simulink model "ADAPT_SDCAL_YesAccum_2Cyl_DA_11_30_2021"  (R2020b)
settings: Solver=ode15s  StartTime=0  StopTime=200  FixedStep=0.00125  MaxStep=0.00125  RelTol=1e-3  EnableMultiTasking=on
values from neighbouring files (symbols this model uses):
  Spring_const = -50    [Four_cyl_design_Param.m]    (also in Four_cyl_design_Param2.m = -200)
  Zero_Spr_F = 4    [Four_cyl_design_Param.m]    (also in Four_cyl_design_Param2.m)
undefined symbols (not defined in the file or in its folder): body, DiscIntNeverNeededParam, geometry, hydroData, pto
libraries: fl_lib x274, nesl_utility x158, sh_lib x128, WECSim_Lib x4
(part 3 of 11)

== system ADAPT_SDCAL_YesAccum_2Cyl_DA_11_30_2021/PTO-Sim - Crankshaft DA 4 Cylinders Case 5 good extra Short cylinders Comp Off/Cylinder 1 ==
  Crank Radius : Inport
  Spool Radius : Inport  Port=2
  Angle Displacement : Inport  Port=3
  Crank Init Angle : Inport  Port=4
  Ext Control Input : Inport  Port=5
  Comp Control Input : Inport  Port=6
  Crank Torque [Nm] : Product
  Crank Torque [Nm] Sensor : Scope
  Cyl1 Force Sensor : Scope
  Cylinder 1 to PTO Force convert : Subsystem
  Hydraulic cylinder and valves : Subsystem
  Ideal Translational Motion Sensor : fl_lib/Mechanical/Mechanical Sensors/Ideal Translational Motion Sensor  offset=0 m
  Mass : fl_lib/Mechanical/Translational Elements/Mass  mass=1 kg  v_specify=off  v_priority=High  v=0 m/s  v_nominal_specify=off  v_nominal_unit=m/s  v_nominal_value=1  f_specify=off  f_priority=None  f=0 N  f_nominal_specify=off  f_nominal_unit=N  f_nominal_value=1
  PTO Force Cyl 1 Sensor : Scope
  Slider-Crank : fl_lib/Mechanical/Mechanisms/Slider-Crank  crank=3.136 in  rod=7 in  inertia=0.01 kg*m^2  k=1e6 N/m  b=0.0001 N/(m/s)  theta_specify=on  theta_priority=High  theta=pi / 2 rad  theta_nominal_specify=off  theta_nominal_unit=rad  theta_nominal_value=1  w_specify=off  w_priority=Low  w=0 rad/s  w_nominal_specify=off  w_nominal_unit=rad/s  w_nominal_value=1
      settings: SourceProductBaseCode=SS  InternalSimscapePortConfiguration="{\"Bottom\":[],\"Left\":[{\"id\":\"C\",\"label\":\"C\",\"type\":\"foundation.mechanical.rotational.rotational\"}],\"Right\":[{\"id\":\"S\",\"label\":\"S\",\"type\":\"foundation.mechanical.translational.translational\"}],\"Top\":[]}"
  Theta sensor : Scope
  sin(theta) sensor : Scope
  Angular Vel Source : PMIOPort  Side=Left
  Flow Out : PMIOPort  Port=2  Side=Left
  Flow In : PMIOPort  Port=3  Side=Left
  PTO Force : Outport
  wires:
  Crank Torque [Nm]/1 -> Crank Torque [Nm] Sensor/1
  Hydraulic cylinder and valves/1(Force Out) -> Cylinder 1 to PTO Force convert/5(Cylinder Force), Cyl1 Force Sensor/1
  Crank Radius/1 -> Cylinder 1 to PTO Force convert/1(Crank radius), Crank Torque [Nm]/1
  Cylinder 1 to PTO Force convert/3(PTO Force Cyl) -> PTO Force/1, Crank Torque [Nm]/2, PTO Force Cyl 1 Sensor/1
  Cylinder 1 to PTO Force convert/2(sing(theta)) -> sin(theta) sensor/1
  Spool Radius/1 -> Cylinder 1 to PTO Force convert/4(Spool radius)
  Cylinder 1 to PTO Force convert/1(Theta) -> Theta sensor/1
  Crank Init Angle/1 -> Cylinder 1 to PTO Force convert/2(Crank initial angle)
  Angle Displacement/1 -> Cylinder 1 to PTO Force convert/3(Angle disp)
  Ext Control Input/1 -> Hydraulic cylinder and valves/1(Ext Control Input)
  Comp Control Input/1 -> Hydraulic cylinder and valves/2(Comp Control Input)
  connections:
  Hydraulic cylinder and valves/LConn1 -- Ideal Translational Motion Sensor/RConn2
  Mass/LConn1 -- Ideal Translational Motion Sensor/RConn1
  Slider-Crank/RConn1 -- Ideal Translational Motion Sensor/LConn1
  Slider-Crank/LConn1 -- Angular Vel Source/RConn1
  Hydraulic cylinder and valves/LConn3 -- Flow In/RConn1
  Hydraulic cylinder and valves/LConn2 -- Flow Out/RConn1

== system ADAPT_SDCAL_YesAccum_2Cyl_DA_11_30_2021/PTO-Sim - Crankshaft DA 4 Cylinders Case 5 good extra Short cylinders Comp Off/Cylinder 2 ==
  Crank Radius : Inport
  Spool Radius : Inport  Port=2
  Angle Displacement : Inport  Port=3
  Crank Init Angle : Inport  Port=4
  Ext Control Input : Inport  Port=5
  Comp Control Input : Inport  Port=6
  Crank Torque [Nm] : Product
  Crank Torque [Nm] Sensor : Scope
  Cyl1 Force Sensor : Scope
  Cylinder 1 to PTO Force convert : Subsystem
  Hydraulic cylinder and valves : Subsystem
  Ideal Translational Motion Sensor : fl_lib/Mechanical/Mechanical Sensors/Ideal Translational Motion Sensor  offset=0 m
  Mass : fl_lib/Mechanical/Translational Elements/Mass  mass=1 kg  v_specify=off  v_priority=High  v=0 m/s  v_nominal_specify=off  v_nominal_unit=m/s  v_nominal_value=1  f_specify=off  f_priority=None  f=0 N  f_nominal_specify=off  f_nominal_unit=N  f_nominal_value=1
  PTO Force Cyl 1 Sensor : Scope
  Slider-Crank : fl_lib/Mechanical/Mechanisms/Slider-Crank  crank=3.136 in  rod=7 in  inertia=0.01 kg*m^2  k=1e6 N/m  b=0.0001 N/(m/s)  theta_specify=on  theta_priority=High  theta=0 rad  theta_nominal_specify=off  theta_nominal_unit=rad  theta_nominal_value=1  w_specify=off  w_priority=Low  w=0 rad/s  w_nominal_specify=off  w_nominal_unit=rad/s  w_nominal_value=1
      settings: SourceProductBaseCode=SS  InternalSimscapePortConfiguration="{\"Bottom\":[],\"Left\":[{\"id\":\"C\",\"label\":\"C\",\"type\":\"foundation.mechanical.rotational.rotational\"}],\"Right\":[{\"id\":\"S\",\"label\":\"S\",\"type\":\"foundation.mechanical.translational.translational\"}],\"Top\":[]}"
  Theta sensor : Scope
  sin(theta) sensor : Scope
  Angular Vel Source : PMIOPort  Side=Left
  Flow Out : PMIOPort  Port=2  Side=Left
  Flow In : PMIOPort  Port=3  Side=Left
  PTO Force : Outport
  wires:
  Crank Torque [Nm]/1 -> Crank Torque [Nm] Sensor/1
  Hydraulic cylinder and valves/1(Force Out) -> Cylinder 1 to PTO Force convert/5(Cylinder Force), Cyl1 Force Sensor/1
  Crank Radius/1 -> Cylinder 1 to PTO Force convert/1(Crank radius), Crank Torque [Nm]/1
  Cylinder 1 to PTO Force convert/3(PTO Force Cyl) -> PTO Force/1, Crank Torque [Nm]/2, PTO Force Cyl 1 Sensor/1
  Cylinder 1 to PTO Force convert/2(sing(theta)) -> sin(theta) sensor/1
  Spool Radius/1 -> Cylinder 1 to PTO Force convert/4(Spool radius)
  Cylinder 1 to PTO Force convert/1(Theta) -> Theta sensor/1
  Crank Init Angle/1 -> Cylinder 1 to PTO Force convert/2(Crank initial angle)
  Angle Displacement/1 -> Cylinder 1 to PTO Force convert/3(Angle disp)
  Ext Control Input/1 -> Hydraulic cylinder and valves/1(Ext Control Input)
  Comp Control Input/1 -> Hydraulic cylinder and valves/2(Comp Control Input)
  connections:
  Hydraulic cylinder and valves/LConn1 -- Ideal Translational Motion Sensor/RConn2
  Mass/LConn1 -- Ideal Translational Motion Sensor/RConn1
  Slider-Crank/RConn1 -- Ideal Translational Motion Sensor/LConn1
  Slider-Crank/LConn1 -- Angular Vel Source/RConn1
  Hydraulic cylinder and valves/LConn3 -- Flow In/RConn1
  Hydraulic cylinder and valves/LConn2 -- Flow Out/RConn1

== system ADAPT_SDCAL_YesAccum_2Cyl_DA_11_30_2021/PTO-Sim - Crankshaft DA 4 Cylinders Case 5 good extra Short cylinders Comp Off/Cylinder 3 ==
  Crank Radius : Inport
  Spool Radius : Inport  Port=2
  Angle Displacement : Inport  Port=3
  Crank Init Angle : Inport  Port=4
  Ext Control Input : Inport  Port=5
  Comp Control Input : Inport  Port=6
  Crank Torque [Nm] : Product
  Crank Torque [Nm] Sensor : Scope
  Cyl1 Force Sensor : Scope
  Cylinder 1 to PTO Force convert : Subsystem
  Hydraulic cylinder and valves : Subsystem
  Ideal Translational Motion Sensor : fl_lib/Mechanical/Mechanical Sensors/Ideal Translational Motion Sensor  offset=0 m
  Mass : fl_lib/Mechanical/Translational Elements/Mass  mass=1 kg  v_specify=off  v_priority=High  v=0 m/s  v_nominal_specify=off  v_nominal_unit=m/s  v_nominal_value=1  f_specify=off  f_priority=None  f=0 N  f_nominal_specify=off  f_nominal_unit=N  f_nominal_value=1
  PTO Force Cyl 1 Sensor : Scope
  Slider-Crank : fl_lib/Mechanical/Mechanisms/Slider-Crank  crank=3.136 in  rod=7 in  inertia=0.01 kg*m^2  k=1e6 N/m  b=0.0001 N/(m/s)  theta_specify=on  theta_priority=High  theta=3*pi/2 rad  theta_nominal_specify=off  theta_nominal_unit=rad  theta_nominal_value=1  w_specify=off  w_priority=Low  w=0 rad/s  w_nominal_specify=off  w_nominal_unit=rad/s  w_nominal_value=1
      settings: SourceProductBaseCode=SS  InternalSimscapePortConfiguration="{\"Bottom\":[],\"Left\":[{\"id\":\"C\",\"label\":\"C\",\"type\":\"foundation.mechanical.rotational.rotational\"}],\"Right\":[{\"id\":\"S\",\"label\":\"S\",\"type\":\"foundation.mechanical.translational.translational\"}],\"Top\":[]}"
  Theta sensor : Scope
  sin(theta) sensor : Scope
  Angular Vel Source : PMIOPort  Side=Left
  Flow Out : PMIOPort  Port=2  Side=Left
  Flow In : PMIOPort  Port=3  Side=Left
  PTO Force : Outport
  wires:
  Crank Torque [Nm]/1 -> Crank Torque [Nm] Sensor/1
  Hydraulic cylinder and valves/1(Force Out) -> Cylinder 1 to PTO Force convert/5(Cylinder Force), Cyl1 Force Sensor/1
  Crank Radius/1 -> Cylinder 1 to PTO Force convert/1(Crank radius), Crank Torque [Nm]/1
  Cylinder 1 to PTO Force convert/3(PTO Force Cyl) -> PTO Force/1, Crank Torque [Nm]/2, PTO Force Cyl 1 Sensor/1
  Cylinder 1 to PTO Force convert/2(sing(theta)) -> sin(theta) sensor/1
  Spool Radius/1 -> Cylinder 1 to PTO Force convert/4(Spool radius)
  Cylinder 1 to PTO Force convert/1(Theta) -> Theta sensor/1
  Crank Init Angle/1 -> Cylinder 1 to PTO Force convert/2(Crank initial angle)
  Angle Displacement/1 -> Cylinder 1 to PTO Force convert/3(Angle disp)
  Ext Control Input/1 -> Hydraulic cylinder and valves/1(Ext Control Input)
  Comp Control Input/1 -> Hydraulic cylinder and valves/2(Comp Control Input)
  connections:
  Hydraulic cylinder and valves/LConn1 -- Ideal Translational Motion Sensor/RConn2
  Mass/LConn1 -- Ideal Translational Motion Sensor/RConn1
  Slider-Crank/RConn1 -- Ideal Translational Motion Sensor/LConn1
  Slider-Crank/LConn1 -- Angular Vel Source/RConn1
  Hydraulic cylinder and valves/LConn3 -- Flow In/RConn1
  Hydraulic cylinder and valves/LConn2 -- Flow Out/RConn1

== system ADAPT_SDCAL_YesAccum_2Cyl_DA_11_30_2021/PTO-Sim - Crankshaft DA 4 Cylinders Case 5 good extra Short cylinders Comp Off/Cylinder 4 ==
  Crank Radius : Inport
  Spool Radius : Inport  Port=2
  Angle Displacement : Inport  Port=3
  Crank Init Angle : Inport  Port=4
  Ext Control Input : Inport  Port=5
  Comp Control Input : Inport  Port=6
  Crank Torque [Nm] : Product
  Crank Torque [Nm] Sensor : Scope
  Cyl1 Force Sensor : Scope
  Cylinder 1 to PTO Force convert : Subsystem
  Hydraulic cylinder and valves : Subsystem
  Ideal Translational Motion Sensor : fl_lib/Mechanical/Mechanical Sensors/Ideal Translational Motion Sensor  offset=0 m
  Mass : fl_lib/Mechanical/Translational Elements/Mass  mass=1 kg  v_specify=off  v_priority=High  v=0 m/s  v_nominal_specify=off  v_nominal_unit=m/s  v_nominal_value=1  f_specify=off  f_priority=None  f=0 N  f_nominal_specify=off  f_nominal_unit=N  f_nominal_value=1
  PTO Force Cyl 1 Sensor : Scope
  Slider-Crank : fl_lib/Mechanical/Mechanisms/Slider-Crank  crank=3.136 in  rod=7 in  inertia=0.01 kg*m^2  k=1e6 N/m  b=0.0001 N/(m/s)  theta_specify=on  theta_priority=High  theta=pi rad  theta_nominal_specify=off  theta_nominal_unit=rad  theta_nominal_value=1  w_specify=off  w_priority=Low  w=0 rad/s  w_nominal_specify=off  w_nominal_unit=rad/s  w_nominal_value=1
      settings: SourceProductBaseCode=SS  InternalSimscapePortConfiguration="{\"Bottom\":[],\"Left\":[{\"id\":\"C\",\"label\":\"C\",\"type\":\"foundation.mechanical.rotational.rotational\"}],\"Right\":[{\"id\":\"S\",\"label\":\"S\",\"type\":\"foundation.mechanical.translational.translational\"}],\"Top\":[]}"
  Theta sensor : Scope
  sin(theta) sensor : Scope
  Angular Vel Source : PMIOPort  Side=Left
  Flow Out : PMIOPort  Port=2  Side=Left
  Flow In : PMIOPort  Port=3  Side=Left
  PTO Force : Outport
  wires:
  Crank Torque [Nm]/1 -> Crank Torque [Nm] Sensor/1
  Hydraulic cylinder and valves/1(Force Out) -> Cylinder 1 to PTO Force convert/5(Cylinder Force), Cyl1 Force Sensor/1
  Crank Radius/1 -> Cylinder 1 to PTO Force convert/1(Crank radius), Crank Torque [Nm]/1
  Cylinder 1 to PTO Force convert/3(PTO Force Cyl) -> PTO Force/1, Crank Torque [Nm]/2, PTO Force Cyl 1 Sensor/1
  Cylinder 1 to PTO Force convert/2(sing(theta)) -> sin(theta) sensor/1
  Spool Radius/1 -> Cylinder 1 to PTO Force convert/4(Spool radius)
  Cylinder 1 to PTO Force convert/1(Theta) -> Theta sensor/1
  Crank Init Angle/1 -> Cylinder 1 to PTO Force convert/2(Crank initial angle)
  Angle Displacement/1 -> Cylinder 1 to PTO Force convert/3(Angle disp)
  Ext Control Input/1 -> Hydraulic cylinder and valves/1(Ext Control Input)
  Comp Control Input/1 -> Hydraulic cylinder and valves/2(Comp Control Input)
  connections:
  Hydraulic cylinder and valves/LConn1 -- Ideal Translational Motion Sensor/RConn2
  Mass/LConn1 -- Ideal Translational Motion Sensor/RConn1
  Slider-Crank/RConn1 -- Ideal Translational Motion Sensor/LConn1
  Slider-Crank/LConn1 -- Angular Vel Source/RConn1
  Hydraulic cylinder and valves/LConn3 -- Flow In/RConn1
  Hydraulic cylinder and valves/LConn2 -- Flow Out/RConn1

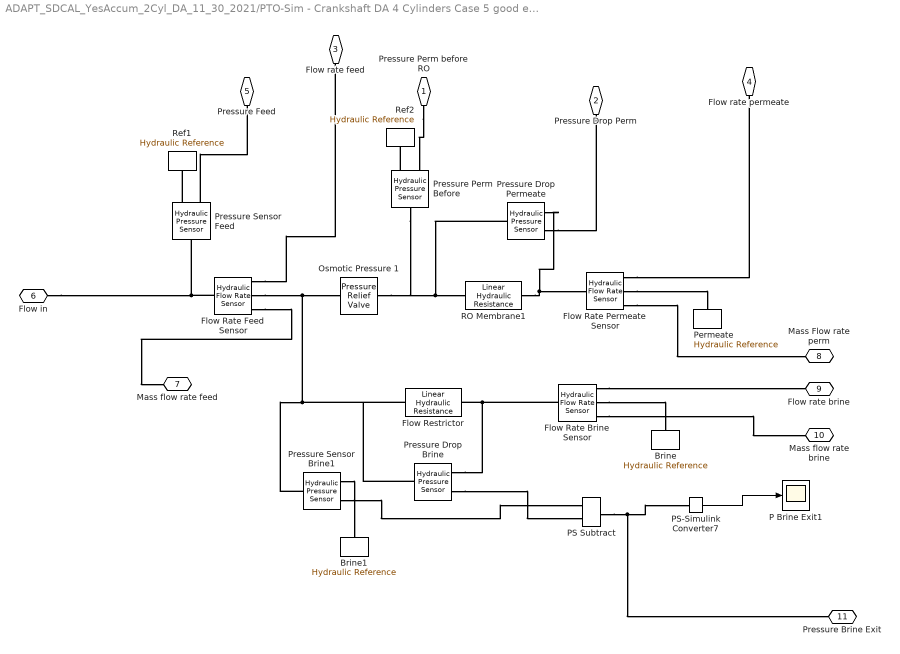
== system ADAPT_SDCAL_YesAccum_2Cyl_DA_11_30_2021/PTO-Sim - Crankshaft DA 4 Cylinders Case 5 good extra Short cylinders Comp Off/RO Membrane ==
  " Flow Rate Feed Sensor" : fl_lib/Hydraulic/Hydraulic Sensors/Hydraulic Flow Rate Sensor
  Brine : fl_lib/Hydraulic/Hydraulic Elements/Hydraulic Reference
  Brine1 : fl_lib/Hydraulic/Hydraulic Elements/Hydraulic Reference
  Flow Rate Brine Sensor : fl_lib/Hydraulic/Hydraulic Sensors/Hydraulic Flow Rate Sensor
  Flow Rate Permeate Sensor : fl_lib/Hydraulic/Hydraulic Sensors/Hydraulic Flow Rate Sensor
  Flow Restrictor : fl_lib/Hydraulic/Hydraulic Elements/Linear Hydraulic Resistance  resistance=(0.90) * ( 1/((3.812*10^-12)*(7.4 ) ) ) Pa/(m^3/s)  q_specify=off  q_priority=None  q=0.001 m^3/s  q_nominal_specify=off  q_nominal_unit=m^3/s  q_nominal_value=1  p_specify=off  p_priority=None  p=0 Pa  p_nominal_specify=off  p_nominal_unit=Pa  p_nominal_value=1
      settings: SourceProductBaseCode=SS  InternalSimscapePortConfiguration="{\"Bottom\":[],\"Left\":[{\"id\":\"A\",\"label\":\"A\",\"type\":\"foundation.hydraulic.hydraulic\"}],\"Right\":[{\"id\":\"B\",\"label\":\"B\",\"type\":\"foundation.hydraulic.hydraulic\"}],\"Top\":[]}"
  Osmotic Pressure 1 : sh_lib/Valves/Pressure Control Valves/Pressure Relief Valve  valve_area_spec=1  p_diff_TLU=[30.15e5 : 15e3 : 31.35e5] Pa  area_TLU=[1 : 1 : 9] .* 1e-5 m^2  area_max=10*pi*(0.75/2)^2 in^2  pres_set=30 bar  reg_range=2 bar  C_d=0.7  A_leak=1e-12 m^2  lam_spec=1  B_lam=0.999  Re_cr=12  dynamic=0  tau=0.1 s  area_init=1e-12 m^2
      settings: SourceProductBaseCode=SH  InternalSimscapePortConfiguration="{\"Bottom\":[],\"Left\":[{\"id\":\"A\",\"label\":\"A\",\"type\":\"foundation.hydraulic.hydraulic\"}],\"Right\":[{\"id\":\"B\",\"label\":\"B\",\"type\":\"foundation.hydraulic.hydraulic\"}],\"Top\":[]}"
  P Brine Exit1 : Scope
  PS Subtract : fl_lib/Physical Signals/Functions/PS Subtract
  PS-Simulink Converter7 : nesl_utility/PS-Simulink Converter  PhysicalDomain=network_engine_domain  SubClassName=ps_output  LeftPortType=input  RightPortType=output  PseudoPeriodic=off  Frequencies=[]  Unit=inherit  AffineConversion=off
  Permeate : fl_lib/Hydraulic/Hydraulic Elements/Hydraulic Reference
  Pressure Drop Brine : fl_lib/Hydraulic/Hydraulic Sensors/Hydraulic Pressure Sensor
  Pressure Drop Permeate : fl_lib/Hydraulic/Hydraulic Sensors/Hydraulic Pressure Sensor
  Pressure Perm Before : fl_lib/Hydraulic/Hydraulic Sensors/Hydraulic Pressure Sensor
  Pressure Sensor Brine1 : fl_lib/Hydraulic/Hydraulic Sensors/Hydraulic Pressure Sensor
  Pressure Sensor Feed : fl_lib/Hydraulic/Hydraulic Sensors/Hydraulic Pressure Sensor
  RO Membrane1 : fl_lib/Hydraulic/Hydraulic Elements/Linear Hydraulic Resistance  resistance=1/((3.812*10^-12)*(7.4 ) ) Pa/(m^3/s)  q_specify=off  q_priority=None  q=0.001 m^3/s  q_nominal_specify=off  q_nominal_unit=m^3/s  q_nominal_value=1  p_specify=off  p_priority=None  p=0 Pa  p_nominal_specify=off  p_nominal_unit=Pa  p_nominal_value=1
      settings: SourceProductBaseCode=SS  InternalSimscapePortConfiguration="{\"Bottom\":[],\"Left\":[{\"id\":\"A\",\"label\":\"A\",\"type\":\"foundation.hydraulic.hydraulic\"}],\"Right\":[{\"id\":\"B\",\"label\":\"B\",\"type\":\"foundation.hydraulic.hydraulic\"}],\"Top\":[]}"
  Ref1 : fl_lib/Hydraulic/Hydraulic Elements/Hydraulic Reference
  Ref2 : fl_lib/Hydraulic/Hydraulic Elements/Hydraulic Reference
  Pressure Perm before RO : PMIOPort  Side=Right
  Pressure Drop Perm : PMIOPort  Port=2  Side=Right
  Flow rate feed : PMIOPort  Port=3  Side=Right
  Flow rate permeate : PMIOPort  Port=4  Side=Right
  Pressure Feed : PMIOPort  Port=5  Side=Right
  Flow in : PMIOPort  Port=6  Side=Left
  Mass flow rate feed : PMIOPort  Port=7  Side=Right
  Mass Flow rate perm : PMIOPort  Port=8  Side=Right
  Flow rate brine : PMIOPort  Port=9  Side=Right
  Mass flow rate brine : PMIOPort  Port=10  Side=Right
  Pressure Brine Exit : PMIOPort  Port=11  Side=Right
  wires:
  PS-Simulink Converter7/1 -> P Brine Exit1/1
  connections:
  RO Membrane1/RConn1 -- Pressure Drop Permeate/RConn1 -- Flow Rate Permeate Sensor/LConn1
  " Flow Rate Feed Sensor"/RConn2 -- Pressure Sensor Brine1/LConn1 -- Pressure Drop Brine/LConn1 -- Flow Restrictor/LConn1 -- Osmotic Pressure 1/LConn1
  Pressure Drop Permeate/LConn1 -- RO Membrane1/LConn1 -- Osmotic Pressure 1/RConn1 -- Pressure Perm Before/LConn1
  Pressure Perm Before/RConn1 -- Ref2/LConn1
  Flow Rate Brine Sensor/LConn1 -- Pressure Drop Brine/RConn1 -- Flow Restrictor/RConn1
  " Flow Rate Feed Sensor"/LConn1 -- Pressure Sensor Feed/LConn1 -- Flow in/RConn1
  Flow Rate Permeate Sensor/RConn2 -- Permeate/LConn1
  Pressure Sensor Brine1/RConn1 -- Brine1/LConn1
  " Flow Rate Feed Sensor"/RConn1 -- Flow rate feed/RConn1
  PS Subtract/RConn1 -- Pressure Brine Exit/RConn1 -- PS-Simulink Converter7/LConn1
  Pressure Sensor Feed/RConn2 -- Pressure Feed/RConn1
  Flow Rate Brine Sensor/RConn2 -- Brine/LConn1
  Pressure Sensor Feed/RConn1 -- Ref1/LConn1
  Flow Rate Permeate Sensor/RConn1 -- Flow rate permeate/RConn1
  Pressure Perm before RO/RConn1 -- Pressure Perm Before/RConn2
  Pressure Drop Brine/RConn2 -- PS Subtract/LConn2
  Pressure Sensor Brine1/RConn2 -- PS Subtract/LConn1
  Pressure Drop Permeate/RConn2 -- Pressure Drop Perm/RConn1
  " Flow Rate Feed Sensor"/RConn3 -- Mass flow rate feed/RConn1
  Flow Rate Permeate Sensor/RConn3 -- Mass Flow rate perm/RConn1
  Flow Rate Brine Sensor/RConn1 -- Flow rate brine/RConn1
  Flow Rate Brine Sensor/RConn3 -- Mass flow rate brine/RConn1

== system ADAPT_SDCAL_YesAccum_2Cyl_DA_11_30_2021/PTO-Sim - Crankshaft DA 4 Cylinders Case 5 good extra Short cylinders Comp Off/Water Quality Block ==
  A_w/Bs : fl_lib/Physical Signals/Functions/PS Gain  gain=3.812*10^(-12)/(6.986*10^(-8))
  C_m : fl_lib/Physical Signals/Sources/PS Constant  constant=35000
  Constant : Constant  Value=0
  Cp : Scope  NumInputPorts=2
  Divide : Product
  If : If
  If Action Perm Flow  > 0 : Subsystem  TreatAsAtomicUnit=on
  If Action Subsystem1 : Subsystem  TreatAsAtomicUnit=on
  P Permeate Exit : Scope
  PS Add : fl_lib/Physical Signals/Functions/PS Add
  PS Constant : fl_lib/Physical Signals/Sources/PS Constant  constant=1 Pa
  PS Divide : fl_lib/Physical Signals/Functions/PS Divide
      settings: SourceProductBaseCode=SS
  PS Subtract1 : fl_lib/Physical Signals/Functions/PS Subtract
  PS-Simulink Converter{5..6,8..11} (6 alike) : nesl_utility/PS-Simulink Converter  PhysicalDomain=network_engine_domain  SubClassName=ps_output  LeftPortType=input  RightPortType=output  PseudoPeriodic=off  Frequencies=[]  Unit=inherit  AffineConversion=off
  Permeate Cp*Flow : Scope
  Recov Ratio : fl_lib/Physical Signals/Functions/PS Divide
      settings: SourceProductBaseCode=SS
  Recov Ratio % : Scope
  Pressure Perm Before : PMIOPort  Side=Left
  Pressure Dop Permeate : PMIOPort  Port=2  Side=Left
  Flow rate feed sensor : PMIOPort  Port=3  Side=Left
  Flow rate permeate : PMIOPort  Port=4  Side=Left
  wires:
  If Action Perm Flow  > 0/1(Out1) -> Cp/2
  Divide/1 -> Permeate Cp*Flow/1
  If/1 -> If Action Perm Flow  > 0/Action
  If Action Subsystem1/1(Out1) -> Cp/1
  If/2 -> If Action Subsystem1/Action
  PS-Simulink Converter10/1 -> Divide/1
  PS-Simulink Converter9/1 -> If/1
  PS-Simulink Converter8/1 -> P Permeate Exit/1
  PS-Simulink Converter6/1 -> Recov Ratio %/1
  PS-Simulink Converter11/1 -> Divide/2
  Constant/1 -> If Action Subsystem1/1(In1)
  PS-Simulink Converter5/1 -> If Action Perm Flow  > 0/1(In1)
  connections:
  A_w/Bs/LConn1 -- PS-Simulink Converter9/LConn1 -- PS Subtract1/LConn1 -- Pressure Perm Before/RConn1
  PS Divide/RConn1 -- PS-Simulink Converter5/LConn1 -- PS-Simulink Converter10/LConn1
  Recov Ratio/RConn1 -- PS-Simulink Converter6/LConn1
  PS Constant/RConn1 -- PS Add/LConn2
  Recov Ratio/LConn1 -- PS-Simulink Converter11/LConn1 -- Flow rate permeate/RConn1
  PS Subtract1/RConn1 -- PS-Simulink Converter8/LConn1
  PS Add/LConn1 -- A_w/Bs/RConn1
  C_m/RConn1 -- PS Divide/LConn1
  PS Divide/LConn2 -- PS Add/RConn1
  Flow rate feed sensor/RConn1 -- Recov Ratio/LConn2
  Pressure Dop Permeate/RConn1 -- PS Subtract1/LConn2

== system ADAPT_SDCAL_YesAccum_2Cyl_DA_11_30_2021/PTO-Sim - Crankshaft DA 4 Cylinders - 1 RO membrane/2 cylinders and valves/Cylinder 1 ==
  Crank Radius : Inport
  Spool Radius : Inport  Port=2
  Angle Displacement : Inport  Port=3
  Crank Init Angle : Inport  Port=4
  Ext Control Input : Inport  Port=5
  Comp Control Input : Inport  Port=6
  Crank Torque [Nm] : Product
  Crank Torque [Nm] Sensor : Scope
  Cyl1 Force Sensor : Scope
  Cylinder 1 to PTO Force convert : Subsystem
  Hydraulic cylinder and valves : Subsystem
  Ideal Translational Motion Sensor : fl_lib/Mechanical/Mechanical Sensors/Ideal Translational Motion Sensor  offset=0 m
  Mass : fl_lib/Mechanical/Translational Elements/Mass  mass=1 kg  num_ports=foundation.enum.numPorts2.one  v_specify=off  v_priority=High  v=0 m/s  v_nominal_specify=off  v_nominal_unit=m/s  v_nominal_value=1  f_specify=off  f_priority=None  f=0 N  f_nominal_specify=off  f_nominal_unit=N  f_nominal_value=1
  PTO Force Cyl 1 Sensor : Scope
  Slider-Crank : fl_lib/Mechanical/Mechanisms/Slider-Crank  crank=3.136 in  rod=7 in  inertia=0.01 kg*m^2  k=1e6 N/m  b=0.0001 N/(m/s)  theta_specify=on  theta_priority=High  theta=pi / 2 rad  theta_nominal_specify=off  theta_nominal_unit=rad  theta_nominal_value=1  w_specify=off  w_priority=Low  w=0 rad/s  w_nominal_specify=off  w_nominal_unit=rad/s  w_nominal_value=1
      settings: SourceProductBaseCode=SS  InternalSimscapePortConfiguration="{\"Bottom\":[],\"Left\":[{\"id\":\"C\",\"label\":\"C\",\"type\":\"foundation.mechanical.rotational.rotational\"}],\"Right\":[{\"id\":\"S\",\"label\":\"S\",\"type\":\"foundation.mechanical.translational.translational\"}],\"Top\":[]}"
  Theta sensor : Scope
  sin(theta) sensor : Scope
  Angular Vel Source : PMIOPort  Side=Left
  Flow Out : PMIOPort  Port=2  Side=Left
  Flow In : PMIOPort  Port=3  Side=Left
  PTO Force : Outport
  wires:
  Crank Torque [Nm]/1 -> Crank Torque [Nm] Sensor/1
  Hydraulic cylinder and valves/1(Force Out) -> Cylinder 1 to PTO Force convert/5(Cylinder Force), Cyl1 Force Sensor/1
  Crank Radius/1 -> Cylinder 1 to PTO Force convert/1(Crank radius), Crank Torque [Nm]/1
  Cylinder 1 to PTO Force convert/3(PTO Force Cyl) -> PTO Force/1, Crank Torque [Nm]/2, PTO Force Cyl 1 Sensor/1
  Cylinder 1 to PTO Force convert/2(sing(theta)) -> sin(theta) sensor/1
  Spool Radius/1 -> Cylinder 1 to PTO Force convert/4(Spool radius)
  Cylinder 1 to PTO Force convert/1(Theta) -> Theta sensor/1
  Crank Init Angle/1 -> Cylinder 1 to PTO Force convert/2(Crank initial angle)
  Angle Displacement/1 -> Cylinder 1 to PTO Force convert/3(Angle disp)
  Ext Control Input/1 -> Hydraulic cylinder and valves/1(Ext Control Input)
  Comp Control Input/1 -> Hydraulic cylinder and valves/2(Comp Control Input)
  connections:
  Hydraulic cylinder and valves/LConn1 -- Ideal Translational Motion Sensor/RConn2
  Mass/LConn1 -- Ideal Translational Motion Sensor/RConn1
  Slider-Crank/RConn1 -- Ideal Translational Motion Sensor/LConn1
  Slider-Crank/LConn1 -- Angular Vel Source/RConn1
  Hydraulic cylinder and valves/LConn3 -- Flow In/RConn1
  Hydraulic cylinder and valves/LConn2 -- Flow Out/RConn1

== system ADAPT_SDCAL_YesAccum_2Cyl_DA_11_30_2021/PTO-Sim - Crankshaft DA 4 Cylinders - 1 RO membrane/2 cylinders and valves/Cylinder 2 ==
  Crank Radius : Inport
  Spool Radius : Inport  Port=2
  Angle Displacement : Inport  Port=3
  Crank Init Angle : Inport  Port=4
  Ext Control Input : Inport  Port=5
  Comp Control Input : Inport  Port=6
  Crank Torque [Nm] : Product
  Crank Torque [Nm] Sensor : Scope
  Cyl1 Force Sensor : Scope
  Cylinder 1 to PTO Force convert : Subsystem
  Hydraulic cylinder and valves : Subsystem
  Ideal Translational Motion Sensor : fl_lib/Mechanical/Mechanical Sensors/Ideal Translational Motion Sensor  offset=0 m
  Mass : fl_lib/Mechanical/Translational Elements/Mass  mass=1 kg  num_ports=foundation.enum.numPorts2.one  v_specify=off  v_priority=High  v=0 m/s  v_nominal_specify=off  v_nominal_unit=m/s  v_nominal_value=1  f_specify=off  f_priority=None  f=0 N  f_nominal_specify=off  f_nominal_unit=N  f_nominal_value=1
  PTO Force Cyl 1 Sensor : Scope
  Slider-Crank : fl_lib/Mechanical/Mechanisms/Slider-Crank  crank=3.136 in  rod=7 in  inertia=0.01 kg*m^2  k=1e6 N/m  b=0.0001 N/(m/s)  theta_specify=on  theta_priority=High  theta=0 rad  theta_nominal_specify=off  theta_nominal_unit=rad  theta_nominal_value=1  w_specify=off  w_priority=Low  w=0 rad/s  w_nominal_specify=off  w_nominal_unit=rad/s  w_nominal_value=1
      settings: SourceProductBaseCode=SS  InternalSimscapePortConfiguration="{\"Bottom\":[],\"Left\":[{\"id\":\"C\",\"label\":\"C\",\"type\":\"foundation.mechanical.rotational.rotational\"}],\"Right\":[{\"id\":\"S\",\"label\":\"S\",\"type\":\"foundation.mechanical.translational.translational\"}],\"Top\":[]}"
  Theta sensor : Scope
  sin(theta) sensor : Scope
  Angular Vel Source : PMIOPort  Side=Left
  Flow Out : PMIOPort  Port=2  Side=Left
  Flow In : PMIOPort  Port=3  Side=Left
  PTO Force : Outport
  wires:
  Crank Torque [Nm]/1 -> Crank Torque [Nm] Sensor/1
  Hydraulic cylinder and valves/1(Force Out) -> Cylinder 1 to PTO Force convert/5(Cylinder Force), Cyl1 Force Sensor/1
  Crank Radius/1 -> Cylinder 1 to PTO Force convert/1(Crank radius), Crank Torque [Nm]/1
  Cylinder 1 to PTO Force convert/3(PTO Force Cyl) -> PTO Force/1, Crank Torque [Nm]/2, PTO Force Cyl 1 Sensor/1
  Cylinder 1 to PTO Force convert/2(sing(theta)) -> sin(theta) sensor/1
  Spool Radius/1 -> Cylinder 1 to PTO Force convert/4(Spool radius)
  Cylinder 1 to PTO Force convert/1(Theta) -> Theta sensor/1
  Crank Init Angle/1 -> Cylinder 1 to PTO Force convert/2(Crank initial angle)
  Angle Displacement/1 -> Cylinder 1 to PTO Force convert/3(Angle disp)
  Ext Control Input/1 -> Hydraulic cylinder and valves/1(Ext Control Input)
  Comp Control Input/1 -> Hydraulic cylinder and valves/2(Comp Control Input)
  connections:
  Hydraulic cylinder and valves/LConn1 -- Ideal Translational Motion Sensor/RConn2
  Mass/LConn1 -- Ideal Translational Motion Sensor/RConn1
  Slider-Crank/RConn1 -- Ideal Translational Motion Sensor/LConn1
  Slider-Crank/LConn1 -- Angular Vel Source/RConn1
  Hydraulic cylinder and valves/LConn3 -- Flow In/RConn1
  Hydraulic cylinder and valves/LConn2 -- Flow Out/RConn1

== system ADAPT_SDCAL_YesAccum_2Cyl_DA_11_30_2021/PTO-Sim - Crankshaft DA 4 Cylinders - 1 RO membrane/2 cylinders and valves/Cylinder 3 ==
  Crank Radius : Inport
  Spool Radius : Inport  Port=2
  Angle Displacement : Inport  Port=3
  Crank Init Angle : Inport  Port=4
  Ext Control Input : Inport  Port=5
  Comp Control Input : Inport  Port=6
  Crank Torque [Nm] : Product
  Crank Torque [Nm] Sensor : Scope
  Cyl1 Force Sensor : Scope
  Cylinder 1 to PTO Force convert : Subsystem
  Hydraulic cylinder and valves : Subsystem
  Ideal Translational Motion Sensor : fl_lib/Mechanical/Mechanical Sensors/Ideal Translational Motion Sensor  offset=0 m
  Mass : fl_lib/Mechanical/Translational Elements/Mass  mass=1 kg  num_ports=foundation.enum.numPorts2.one  v_specify=off  v_priority=High  v=0 m/s  v_nominal_specify=off  v_nominal_unit=m/s  v_nominal_value=1  f_specify=off  f_priority=None  f=0 N  f_nominal_specify=off  f_nominal_unit=N  f_nominal_value=1
  PTO Force Cyl 1 Sensor : Scope
  Slider-Crank : fl_lib/Mechanical/Mechanisms/Slider-Crank  crank=3.136 in  rod=7 in  inertia=0.01 kg*m^2  k=1e6 N/m  b=0.0001 N/(m/s)  theta_specify=on  theta_priority=High  theta=3*pi/2 rad  theta_nominal_specify=off  theta_nominal_unit=rad  theta_nominal_value=1  w_specify=off  w_priority=Low  w=0 rad/s  w_nominal_specify=off  w_nominal_unit=rad/s  w_nominal_value=1
      settings: SourceProductBaseCode=SS  InternalSimscapePortConfiguration="{\"Bottom\":[],\"Left\":[{\"id\":\"C\",\"label\":\"C\",\"type\":\"foundation.mechanical.rotational.rotational\"}],\"Right\":[{\"id\":\"S\",\"label\":\"S\",\"type\":\"foundation.mechanical.translational.translational\"}],\"Top\":[]}"
  Theta sensor : Scope
  sin(theta) sensor : Scope
  Angular Vel Source : PMIOPort  Side=Left
  Flow Out : PMIOPort  Port=2  Side=Left
  Flow In : PMIOPort  Port=3  Side=Left
  PTO Force : Outport
  wires:
  Crank Torque [Nm]/1 -> Crank Torque [Nm] Sensor/1
  Hydraulic cylinder and valves/1(Force Out) -> Cylinder 1 to PTO Force convert/5(Cylinder Force), Cyl1 Force Sensor/1
  Crank Radius/1 -> Cylinder 1 to PTO Force convert/1(Crank radius), Crank Torque [Nm]/1
  Cylinder 1 to PTO Force convert/3(PTO Force Cyl) -> PTO Force/1, Crank Torque [Nm]/2, PTO Force Cyl 1 Sensor/1
  Cylinder 1 to PTO Force convert/2(sing(theta)) -> sin(theta) sensor/1
  Spool Radius/1 -> Cylinder 1 to PTO Force convert/4(Spool radius)
  Cylinder 1 to PTO Force convert/1(Theta) -> Theta sensor/1
  Crank Init Angle/1 -> Cylinder 1 to PTO Force convert/2(Crank initial angle)
  Angle Displacement/1 -> Cylinder 1 to PTO Force convert/3(Angle disp)
  Ext Control Input/1 -> Hydraulic cylinder and valves/1(Ext Control Input)
  Comp Control Input/1 -> Hydraulic cylinder and valves/2(Comp Control Input)
  connections:
  Hydraulic cylinder and valves/LConn1 -- Ideal Translational Motion Sensor/RConn2
  Mass/LConn1 -- Ideal Translational Motion Sensor/RConn1
  Slider-Crank/RConn1 -- Ideal Translational Motion Sensor/LConn1
  Slider-Crank/LConn1 -- Angular Vel Source/RConn1
  Hydraulic cylinder and valves/LConn3 -- Flow In/RConn1
  Hydraulic cylinder and valves/LConn2 -- Flow Out/RConn1

== system ADAPT_SDCAL_YesAccum_2Cyl_DA_11_30_2021/PTO-Sim - Crankshaft DA 4 Cylinders - 1 RO membrane/2 cylinders and valves/Cylinder 4 ==
  Crank Radius : Inport
  Spool Radius : Inport  Port=2
  Angle Displacement : Inport  Port=3
  Crank Init Angle : Inport  Port=4
  Ext Control Input : Inport  Port=5
  Comp Control Input : Inport  Port=6
  Crank Torque [Nm] : Product
  Crank Torque [Nm] Sensor : Scope
  Cyl1 Force Sensor : Scope
  Cylinder 1 to PTO Force convert : Subsystem
  Hydraulic cylinder and valves : Subsystem
  Ideal Translational Motion Sensor : fl_lib/Mechanical/Mechanical Sensors/Ideal Translational Motion Sensor  offset=0 m
  Mass : fl_lib/Mechanical/Translational Elements/Mass  mass=1 kg  num_ports=foundation.enum.numPorts2.one  v_specify=off  v_priority=High  v=0 m/s  v_nominal_specify=off  v_nominal_unit=m/s  v_nominal_value=1  f_specify=off  f_priority=None  f=0 N  f_nominal_specify=off  f_nominal_unit=N  f_nominal_value=1
  PTO Force Cyl 1 Sensor : Scope
  Slider-Crank : fl_lib/Mechanical/Mechanisms/Slider-Crank  crank=3.136 in  rod=7 in  inertia=0.01 kg*m^2  k=1e6 N/m  b=0.0001 N/(m/s)  theta_specify=on  theta_priority=High  theta=pi rad  theta_nominal_specify=off  theta_nominal_unit=rad  theta_nominal_value=1  w_specify=off  w_priority=Low  w=0 rad/s  w_nominal_specify=off  w_nominal_unit=rad/s  w_nominal_value=1
      settings: SourceProductBaseCode=SS  InternalSimscapePortConfiguration="{\"Bottom\":[],\"Left\":[{\"id\":\"C\",\"label\":\"C\",\"type\":\"foundation.mechanical.rotational.rotational\"}],\"Right\":[{\"id\":\"S\",\"label\":\"S\",\"type\":\"foundation.mechanical.translational.translational\"}],\"Top\":[]}"
  Theta sensor : Scope
  sin(theta) sensor : Scope
  Angular Vel Source : PMIOPort  Side=Left
  Flow Out : PMIOPort  Port=2  Side=Left
  Flow In : PMIOPort  Port=3  Side=Left
  PTO Force : Outport
  wires:
  Crank Torque [Nm]/1 -> Crank Torque [Nm] Sensor/1
  Hydraulic cylinder and valves/1(Force Out) -> Cylinder 1 to PTO Force convert/5(Cylinder Force), Cyl1 Force Sensor/1
  Crank Radius/1 -> Cylinder 1 to PTO Force convert/1(Crank radius), Crank Torque [Nm]/1
  Cylinder 1 to PTO Force convert/3(PTO Force Cyl) -> PTO Force/1, Crank Torque [Nm]/2, PTO Force Cyl 1 Sensor/1
  Cylinder 1 to PTO Force convert/2(sing(theta)) -> sin(theta) sensor/1
  Spool Radius/1 -> Cylinder 1 to PTO Force convert/4(Spool radius)
  Cylinder 1 to PTO Force convert/1(Theta) -> Theta sensor/1
  Crank Init Angle/1 -> Cylinder 1 to PTO Force convert/2(Crank initial angle)
  Angle Displacement/1 -> Cylinder 1 to PTO Force convert/3(Angle disp)
  Ext Control Input/1 -> Hydraulic cylinder and valves/1(Ext Control Input)
  Comp Control Input/1 -> Hydraulic cylinder and valves/2(Comp Control Input)
  connections:
  Hydraulic cylinder and valves/LConn1 -- Ideal Translational Motion Sensor/RConn2
  Mass/LConn1 -- Ideal Translational Motion Sensor/RConn1
  Slider-Crank/RConn1 -- Ideal Translational Motion Sensor/LConn1
  Slider-Crank/LConn1 -- Angular Vel Source/RConn1
  Hydraulic cylinder and valves/LConn3 -- Flow In/RConn1
  Hydraulic cylinder and valves/LConn2 -- Flow Out/RConn1

== system ADAPT_SDCAL_YesAccum_2Cyl_DA_11_30_2021/PTO-Sim - Crankshaft DA 4 Cylinders - 1 RO membrane/Water Quality Block/If Action Perm Flow  > 0 ==
  In1 : Inport
  Action Port : ActionPort  ActionPortLabel=if(u1 > 0)
  Out1 : Outport
  wires:
  In1/1 -> Out1/1

== system ADAPT_SDCAL_YesAccum_2Cyl_DA_11_30_2021/PTO-Sim - Crankshaft DA 4 Cylinders - 1 RO membrane/Water Quality Block/If Action Subsystem1 ==
  In1 : Inport
  Action Port : ActionPort  ActionPortLabel=else
  Out1 : Outport
  wires:
  In1/1 -> Out1/1

== system ADAPT_SDCAL_YesAccum_2Cyl_DA_11_30_2021/PTO-Sim - Crankshaft DA 4 Cylinders Case 1 good extra/Cylinder 1/Cylinder 1 to PTO Force convert ==
  Crank radius : Inport
  Crank initial angle : Inport  Port=2
  Angle disp : Inport  Port=3
  Spool radius : Inport  Port=4
  Cylinder Force : Inport  Port=5
  Constant : Constant
  Divide1 : Product  Inputs=*/
  Mod angle : Constant  Value=2*pi
  PTO Force Cylinder 1 : Product  Inputs=4
  Sin(theta) : Trigonometry
  Sum : Sum  Inputs=|++
  To get Theta : Math  Operator=mod  SaturateOnIntegerOverflow=on
  Theta : Outport
  sing(theta) : Outport  Port=2
  PTO Force Cyl : Outport  Port=3
  wires:
  Mod angle/1 -> To get Theta/2
  Angle disp/1 -> Sum/2
  To get Theta/1 -> Theta/1, Sin(theta)/1
  PTO Force Cylinder 1/1 -> PTO Force Cyl/1
  Divide1/1 -> PTO Force Cylinder 1/3
  Sin(theta)/1 -> sing(theta)/1, PTO Force Cylinder 1/2
  Constant/1 -> Divide1/1
  Crank initial angle/1 -> Sum/1
  Sum/1 -> To get Theta/1
  Spool radius/1 -> Divide1/2
  Cylinder Force/1 -> PTO Force Cylinder 1/4
  Crank radius/1 -> PTO Force Cylinder 1/1
